simulink model "IdentificacionSimulink"  (R2020a)
settings: Solver=VariableStepAuto  StartTime=0.0  StopTime=15  RelTol=1e-3
libraries: simulink x1
settings Model: Creator=HP  LastModifiedBy=HP

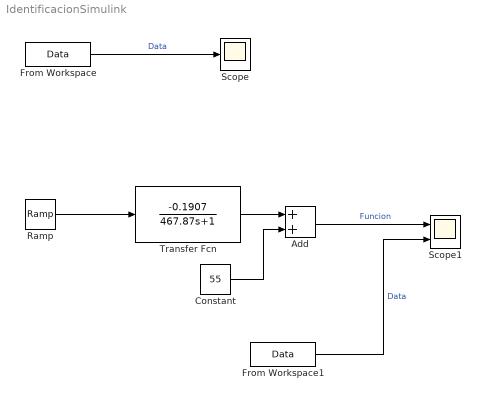
== system IdentificacionSimulink ==
  Add : Sum
  Constant : Constant  Value=55
  From Workspace : FromWorkspace  VariableName=Data
  From Workspace1 : FromWorkspace  VariableName=Data
  Ramp : simulink/Sources/Ramp  slope=1  start=0  InitialOutput=0
  Scope : Scope
  Scope1 : Scope  NumInputPorts=2
  Transfer Fcn : TransferFcn  Numerator=[-0.1907]  Denominator=[467.87 1]
  wires:
  From Workspace/1 -> Scope/1  "Data"
  Ramp/1 -> Transfer Fcn/1
  From Workspace1/1 -> Scope1/2  "Data"
  Transfer Fcn/1 -> Add/1
  Add/1 -> Scope1/1  "Funcion"
  Constant/1 -> Add/2
